simulink model "zbiornik_sys"  (R2021b)
settings: Solver=ode45  StartTime=0.0  StopTime=10.0  RelTol=1e-3
values from neighbouring files (symbols this model uses):
  T0 = 293    [nieliniowy.m]    (also in stan_ustalony.m)
  V0 = 0.04    [nieliniowy.m]    (also in stan_ustalony.m)
settings Model: Creator=Michał  LastModifiedBy=jpawl
settings SolverCC: AlgebraicLoopSolver=TrustRegion
settings DataIOCC: LimitDataPoints=on  SaveFormat=Array  SignalLoggingSaveFormat=ModelDataLogs  ReturnWorkspaceOutputs=off
settings OptimizationCC: BlockReduction=off  BooleanDataType=off  ExpressionDepthLimit=2147483647  LifeSpan=inf
settings DebuggingCC: SaveWithParameterizedLinksMsg=none  UnderspecifiedInitializationDetection=Classic  MergeDetectMultiDrivingBlocksExec=none  SignalResolutionControl=TryResolveAllWithWarning  MultiTaskDSMMsg=warning  MultiTaskCondExecSysMsg=none  StateNameClashWarn=warning  SFUnexpectedBacktrackingDiag=warning  SFNoUnconditionalDefaultTransitionDiag=warning  SFExecutionAtInitializationDiag=none  SFMachineParentedDataDiag=warning  ArithmeticOperatorsInVariantConditions=warning
settings HardwareCC: ProdBitPerPointer=32  ProdBitPerSizeT=32  ProdBitPerPtrDiffT=32  ProdLargestAtomicFloat=None  ProdIntDivRoundTo=Undefined  ProdEndianess=Unspecified  ProdWordSize=32  ProdHWDeviceType=32-bit Generic  TargetUnknown=on
settings ModelReferenceCC: PropagateSignalLabelsOutOfModel=off
settings SFSimCC: SimUseLocalCustomCode=off  CustomCodeUndefinedFunction=UseInterfaceOnly
settings RTWCC: RTWUseLocalCustomCode=off
settings CodeAppCC: StateflowObjectComments=on
settings GRTTargetCC: TargetLangStandard=C89/C90 (ANSI)
settings ConfigComp: CovMetricSettings=dw  CovSaveCumulativeToWorkspaceVar=on  CovSaveSingleToWorkspaceVar=on  CovExternalEMLEnable=off

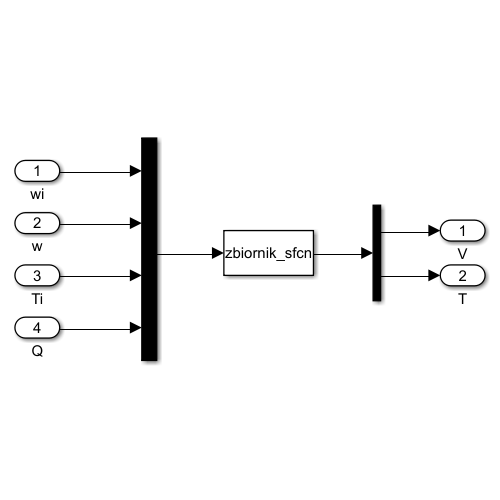
[thumbnail: Simulink's stored preview of the top-level diagram]
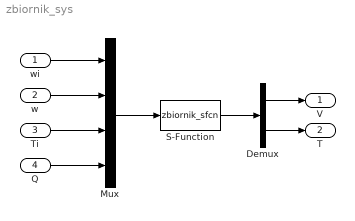
== system zbiornik_sys ==
  wi : Inport
  w : Inport  Port=2
  Ti : Inport  Port=3
  Q : Inport  Port=4
  Demux : Demux  Outputs=2
  Mux : Mux
  S-Function : S-Function  FunctionName=zbiornik_sfcn  Parameters=V0 T0  SFunctionDeploymentMode=off  EnableBusSupport=off
  V : Outport
  T : Outport  Port=2
  wires:
  wi/1 -> Mux/1
  w/1 -> Mux/2
  Ti/1 -> Mux/3
  Q/1 -> Mux/4
  Mux/1 -> S-Function/1
  Demux/2 -> T/1
  S-Function/1 -> Demux/1
  Demux/1 -> V/1
